simulink model "NataliaQAM16"  (Simulink 7.5)
settings: Solver=ode45  StartTime=0.0  StopTime=0.003  RelTol=1e-3
undefined symbols (not defined in the file or in its folder): CRC, Fs, get, Iter, Len, Max, sided, Two, Variance
libraries: dspobslib x6, commsequence2 x6, commblkintrlv2 x6, dspindex x5, commcnvcod2 x4, commcrc2 x2, commdigbbndam3 x2, dspsnks4 x2, dspxfrm3 x2, dspsigops x2, commseqgen2 x2, commutil2 x2
settings Model: Creator=Natalia  LastModifiedBy=Natalia

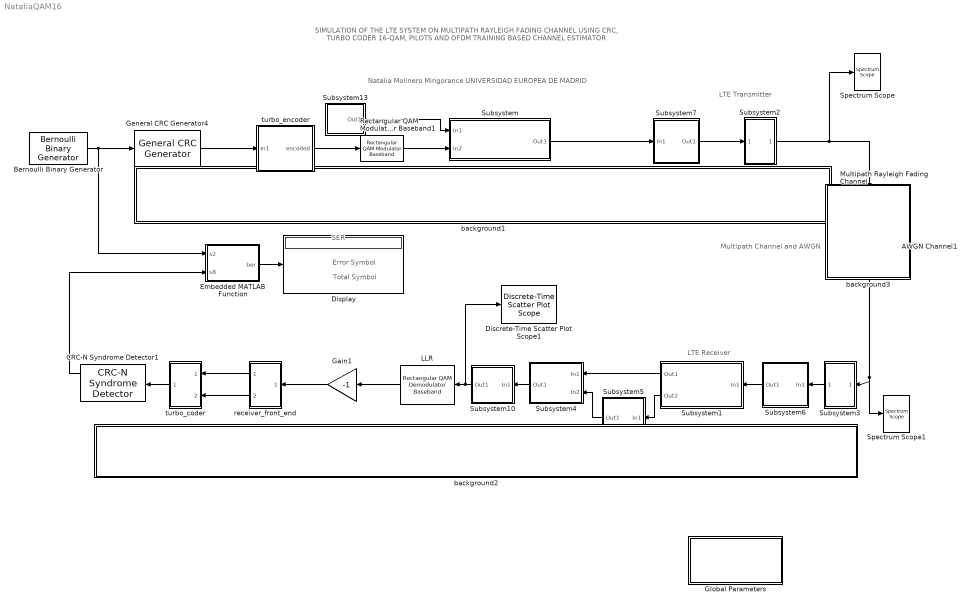
== system NataliaQAM16 ==
  note: SER
  note: Error Symbol
  note: Total Symbol
  note: SIMULATION OF THE LTE SYSTEM ON MULTIPATH RAYLEIGH FADING CHANNEL
      | USING CRC, TURBO CODER 16-QAM, PILOTS AND OFDM
      | TRAINING BASED CHANNEL ESTIMATOR
  note: Natalia Molinero Mingorance
      | UNIVERSIDAD EUROPEA DE MADRID
  note: LTE Transmitter
  note: LTE Receiver
  note: Multipath Channel
      | and AWGN
  AWGN Channel1 : commchan3/AWGN Channel  SystemSampleTime=-1  seed=32965  noiseMode="Signal to noise ratio  (Es/No)"  EbNodB=10  EsNodB=5  SNRdB=0  bitsPerSym=1  Ps=30/(5.5e5*11/15*2.4)*1.08  Tsym=80e-6  variance=1
  Bernoulli Binary Generator : commrandsrc2/Bernoulli Binary Generator  DialogController=commDDGCreate  DialogControllerArgs=DataTag0  SystemSampleTime=-1  P=0.5  seed=61  Ts=1  frameBased=on  sampPerFrame=20  orient=off  outDataType=boolean
  CRC-N Syndrome Detector1 : commcrc2/CRC-N Syndrome Detector  SystemSampleTime=-1  crcMethod=CRC-24  iniStates=[0]  numChecksums=1
  Discrete-Time Scatter Plot Scope1 : commsink2/Discrete-Time Scatter Plot Scope  Tag=ScatterPlot  SystemSampleTime=-1  sampPerSymb=1  offsetEye=0  numTraces=40  numNewFrames=10  LineMarkers=.  LineColors=b  fading=on  render=on  AxisGrid=on  xMin=-0.707933120701309  xMax=0.713103512853537  yMin=-0.710699489007895  yMax=0.71033714454695  inphaseLabel=In-phase Amplitude  quadratureLabel=Quadrature Amplitude  openScopeAtSimStart=on  FrameNumber=off  FigPos=get(0,'defaultfigureposition');  figTitle=Scatter Plot  numLinesMax=8  block_type_=scatter
  Display : Display
  Embedded MATLAB Function : Stateflow chart  TreatAsAtomicUnit=on
  Gain1 : Gain  Gain=-1  SaturateOnIntegerOverflow=on  OutDataTypeStr=Inherit: Same as input  ParamDataTypeStr=Inherit: Same as input
  General CRC Generator4 : commcrc2/General CRC Generator  genPoly=[24,23,6,5,1,0]  iniStates=[0]  numChecksums=1
  Global Parameters : Subsystem  mask(Global Parameters){EbNodB=11, Len=44, Iter=5, Seed=54123}
      mask prompts: EbNodB "Eb/No in dB:"; Len "Block size:"; Iter "Number of iterations:"
      mask help: Load global parameters in MATLAB workspace.
      mask init:
      | turbo_code_punc_setup;
      mask CallbackString: turbo_code_setup;|turbo_code_setup|turbo_code_setup;|turbo_code_setup;
      mask Display: disp(['Eb/No ' num2str(EbNodB,'%3.1f') 'dB'  sprintf('\n') 'Block size   ' num2str(Len,'%7.0f')  sprintf('\n') 'Iterations   ' num2str(Iter,'%3.0f')   sprintf('\n') 'Seed   ' num2str(Seed,'%7.0f')])
  LLR : commdigbbndam3/Rectangular QAM Demodulator Baseband  DialogController=commDDGCreate  DialogControllerArgs=DataTag1  M=16  PowType=Average Power  MinDist=2  AvgPow=0.5  PeakPow=1  Ph=0  Dec=Gray  Mapping=[0:15]  OutType=Bit  DecType=Log-likelihood ratio  VarSource=Dialog  Variance=Variance  outDtype1=double  outDtype2=double  derotateFactorWordLen=16  denormFactorWordLen=16  prodOutWordLen=32  prodOutRoundingMode=Floor  prodOutOverflowMode=Wrap  sumWordLen=32
  Multipath Rayleigh Fading Channel : commchan2/Multipath Rayleigh Fading Channel  SystemSampleTime=-1  Fd=299  simTs=8e-5/180  delayVec=[0 3e-6]  gainVecdB=[0 8]  normGain=on  Seed=936497248
  Rectangular QAM Modulator Baseband1 : commdigbbndam3/Rectangular QAM Modulator Baseband  DialogController=commDDGCreate  DialogControllerArgs=DataTag2  M=16  InType=Bit  Enc=Gray  Mapping=[0:15]  PowType=Average Power  MinDist=2  AvgPow=0.5  PeakPow=1  Ph=0  outDtype=double  outWordLen=16  outUDDataType=sfix(16)  outFracLenMode=Best precision  outFracLen=15
  Spectrum Scope : dspsnks4/Spectrum Scope  DialogController=dspdialog.SpectrumScope  DialogControllerArgs=DataTag3  SystemSampleTime=-1  ScopeProperties=on  Domain=Frequency  HorizSpan=1  UseBuffer=on  BufferSize=90  Overlap=64  inpFftLenInherit=on  FFTlength=1024  numAvg=16  DisplayProperties=off  AxisGrid=on  Memory=off  FrameNumber=on  AxisLegend=off  AxisZoom=off  OpenScopeAtSimStart=on  OpenScopeImmediately=off  FigPos=get(0,'defaultfigureposition')  AxisProperties=off  XUnits=Hertz  XRange=Two-sided ((-Fs/2...Fs/2])  XDisplay=0  InheritXIncr=on  XIncr=1.0  XLabel=Samples  XLimit=Auto  YUnits=dBW/Hertz  XMax=1  XMin=0  YLabel=Magnitude-squared, dB  LineProperties=off  wintypeSpecScope=Hann  RsSpecScope=50  betaSpecScope=5  winsampSpecScope=Periodic  XAxisParamsVer=6.9
      settings: YMin=-10  YMax=10
  Spectrum Scope1 : dspsnks4/Spectrum Scope  DialogController=dspdialog.SpectrumScope  DialogControllerArgs=DataTag4  SystemSampleTime=-1  ScopeProperties=on  Domain=Frequency  HorizSpan=1  UseBuffer=on  BufferSize=90  Overlap=64  inpFftLenInherit=on  FFTlength=1024  numAvg=16  DisplayProperties=off  AxisGrid=on  Memory=off  FrameNumber=on  AxisLegend=off  AxisZoom=off  OpenScopeAtSimStart=on  OpenScopeImmediately=off  FigPos=get(0,'defaultfigureposition')  AxisProperties=off  XUnits=Hertz  XRange=Two-sided ((-Fs/2...Fs/2])  XDisplay=0  InheritXIncr=on  XIncr=1.0  XLabel=Samples  XLimit=Auto  YUnits=dBW/Hertz  XMax=1  XMin=0  YLabel=Magnitude-squared, dB  LineProperties=off  wintypeSpecScope=Hann  RsSpecScope=50  betaSpecScope=5  winsampSpecScope=Periodic  XAxisParamsVer=6.9
      settings: YMin=-10  YMax=10
  Subsystem : Subsystem
      mask Display: disp('OFDM Baseband\nModulator\ndan\nAdd Cyclic Prefix')
  Subsystem1 : Subsystem
      mask Display: disp('OFDM Baseband\nDemodulator\ndan \nRemove Cyclic prefix')
  Subsystem10 : Subsystem
      mask Display: disp('Remove\nZero')
  Subsystem13 : Subsystem
      mask Display: disp('Training')
  Subsystem2 : Subsystem
      mask Display: disp('P/S')
  Subsystem3 : Subsystem
      mask Display: disp('S/P')
  Subsystem4 : Subsystem
      mask Display: disp('Channel\nCompensation')
  Subsystem5 : Subsystem
      mask Display: disp('Channel\nEstimator')
  Subsystem6 : Subsystem
      mask Display: disp('Training\nSeparation')
  Subsystem7 : Subsystem
      mask Display: disp('Training\nInsertion')
  background1 : Subsystem
      mask Display: disp('')
  background2 : Subsystem
      mask Display: disp('')
  background3 : Subsystem
      mask Display: disp('')
  receiver_front_end : Subsystem
  turbo_coder : Subsystem
  turbo_encoder : Subsystem
  wires:
  receiver_front_end/1(Out1) -> turbo_coder/1(In1)
  receiver_front_end/2(Out2) -> turbo_coder/2(In2)
  turbo_encoder/1(encoded) -> Rectangular QAM Modulator Baseband1/1
  LLR/1 -> Gain1/1
  Gain1/1 -> receiver_front_end/1(In1)
  Subsystem13/1(Out1) -> Subsystem/1(In1)
  Subsystem/1(Out1) -> Subsystem7/1(In1)
  Subsystem7/1(Out1) -> Subsystem2/1(In1)
  Rectangular QAM Modulator Baseband1/1 -> Subsystem/2(In2)
  Subsystem1/1(Out1) -> Subsystem4/1(In1)
  Subsystem1/2(Out2) -> Subsystem5/1(In1)
  Subsystem5/1(Out1) -> Subsystem4/2(In2)
  Subsystem4/1(Out1) -> Subsystem10/1(In1)
  Subsystem6/1(Out1) -> Subsystem1/1(In1)
  Subsystem3/1(Out1) -> Subsystem6/1(In1)
  Subsystem10/1(Out1) -> LLR/1, Discrete-Time Scatter Plot Scope1/1
  Multipath Rayleigh Fading Channel/1 -> AWGN Channel1/1
  AWGN Channel1/1 -> Subsystem3/1(In1), Spectrum Scope1/1
  Subsystem2/1(Out1) -> Multipath Rayleigh Fading Channel/1, Spectrum Scope/1
  General CRC Generator4/1 -> turbo_encoder/1(In1)
  turbo_coder/1(Out1) -> CRC-N Syndrome Detector1/1
  Embedded MATLAB Function/1(ber) -> Display/1
  Bernoulli Binary Generator/1 -> General CRC Generator4/1, Embedded MATLAB Function/1(s2)
  CRC-N Syndrome Detector1/1 -> Embedded MATLAB Function/2(s8)

== system NataliaQAM16/Global Parameters ==

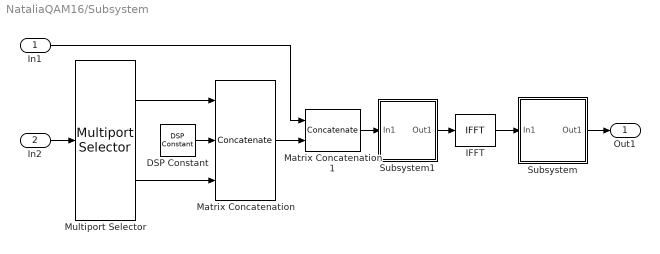
== system NataliaQAM16/Subsystem ==
  In1 : Inport  OutDataType=sfix(16)  OutScaling=2^0
  In2 : Inport  Port=2  OutDataType=sfix(16)  OutScaling=2^0
  DSP Constant : dspobslib/DSP Constant  SystemSampleTime=-1  Value=0  SampleMode=Discrete  discreteOutput=Frame-based  continuousOutput=Sample-based  sampTime=16e-5/2  framePeriod=16e-5/2  dataType=Inherit from 'Constant value'  isSigned=on  wordLen=16  udDataType=sfix(16)  fracBitsMode=Best precision  numFracBits=15  InterpretAs1D=off  Ts=16e-5/2  FramebasedOutput=on
  IFFT : dspxfrm3/IFFT  DialogController=dspDDGCreate  DialogControllerArgs=DataTag5  CompMethod=Table lookup  TableOpt=HYBRID  TableOptActive=Speed  BitRevOrder=off  cs_in=off  SkipNorm=on  InheritFFTLength=on  FFTLength=64  mode=Real  outSamplingMode=Frame based  firstCoeffDataTypeStr=Inherit: Same word length as input  firstCoeffLastDataTypeStr=Inherit: Same word length as input  outputMin=[]  outputMax=[]  roundingMode=Floor  overflowMode=off
  Matrix Concatenation : Concatenate  NumInputs=3  Mode=Multidimensional array
  Matrix Concatenation1 : Concatenate  Mode=Multidimensional array  ConcatenateDimension=2
  Multiport Selector : dspindex/Multiport Selector  rowsOrCols=Rows  idxCellArray={1:11,12:22}  idxErrMode=Clip Index
  Subsystem : Subsystem
      mask Display: disp('Add\nCyclic Prefix')
  Subsystem1 : Subsystem
      mask Display: disp('Zero Pad')
  Out1 : Outport
  wires:
  IFFT/1 -> Subsystem/1(In1)
  Multiport Selector/1 -> Matrix Concatenation/1
  Multiport Selector/2 -> Matrix Concatenation/3
  DSP Constant/1 -> Matrix Concatenation/2
  Subsystem1/1(Out1) -> IFFT/1
  Subsystem/1(Out1) -> Out1/1
  In2/1 -> Multiport Selector/1
  Matrix Concatenation1/1 -> Subsystem1/1(In1)
  Matrix Concatenation/1 -> Matrix Concatenation1/2
  In1/1 -> Matrix Concatenation1/1

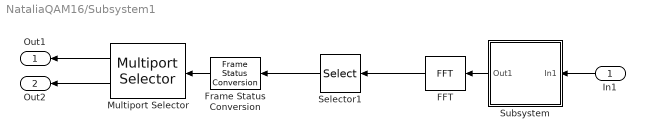
== system NataliaQAM16/Subsystem1 ==
  In1 : Inport  OutDataType=sfix(16)  OutScaling=2^0
  FFT : dspxfrm3/FFT  DialogController=dspDDGCreate  DialogControllerArgs=DataTag6  CompMethod=Table lookup  TableOpt=HYBRID  TableOptActive=Speed  BitRevOrder=off  InheritFFTLength=on  FFTLength=64  SkipNorm=on  firstCoeffDataTypeStr=Inherit: Same word length as input  firstCoeffLastDataTypeStr=Inherit: Same word length as input  outputMin=[]  outputMax=[]  roundingMode=Floor  overflowMode=off
  Frame Status Conversion : dspobslib/Frame Status Conversion  SystemSampleTime=-1  growRefPort=off  outframe=Frame-based
  Multiport Selector : dspindex/Multiport Selector  rowsOrCols=Columns  idxCellArray={1,2}  idxErrMode=Clip Index
  Selector1 : Selector  NumberOfDimensions=2  InputPortWidth=64  IndexOptions=Index vector (dialog),Select all  Indices=[54:64,1:12],-1  OutputSizes=1
  Subsystem : Subsystem
      mask Display: disp('Remove\nCyclic Prefix')
  Out1 : Outport
  Out2 : Outport  Port=2
  wires:
  FFT/1 -> Selector1/1
  Selector1/1 -> Frame Status Conversion/1
  Subsystem/1(Out1) -> FFT/1
  In1/1 -> Subsystem/1(In1)
  Frame Status Conversion/1 -> Multiport Selector/1
  Multiport Selector/1 -> Out1/1
  Multiport Selector/2 -> Out2/1

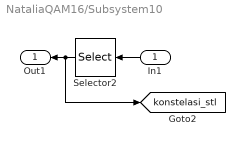
== system NataliaQAM16/Subsystem10 ==
  In1 : Inport  OutDataType=sfix(16)  OutScaling=2^0
  Selector2 : Selector  NumberOfDimensions=2  InputPortWidth=31  IndexOptions=Index vector (dialog),Select all  Indices=[1:11,13:23],-1  OutputSizes=1
  Out1 : Outport
  tag scope: konstelasi_stl=global
  wires:
  Selector2/1 -> Out1/1, [konstelasi_stl]
  In1/1 -> Selector2/1

== system NataliaQAM16/Subsystem13 ==
  PN Sequence Generator : commseqgen2/PN Sequence Generator  poly=[1 0 0 0 0 1 1]  ini_sta=[0 0 0 0 0 1]  outBitMaskSource=Dialog parameter  shift=0  Ts=16e-5/2/23  frameBased=on  sampPerFrame=23  reset=off  bitPackedOutputs=off  outDataType=double  numPackedBits=8  bitPackDataSigned=off  bitPackedOutDType=double
  Unipolar to Bipolar Converter : commutil2/Unipolar to Bipolar Converter  SystemSampleTime=-1  M=2  polarity=Positive  dataType=Inherit via internal rule
  Out1 : Outport
  wires:
  PN Sequence Generator/1 -> Unipolar to Bipolar Converter/1
  Unipolar to Bipolar Converter/1 -> Out1/1

== system NataliaQAM16/Subsystem2 ==
  In1 : Inport  OutDataType=sfix(16)  OutScaling=2^0
  Unbuffer3 : dspbuff3/Unbuffer  ic=0
  Out1 : Outport
  wires:
  In1/1 -> Unbuffer3/1
  Unbuffer3/1 -> Out1/1

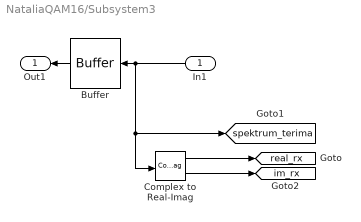
== system NataliaQAM16/Subsystem3 ==
  In1 : Inport  OutDataType=sfix(16)  OutScaling=2^0
  Buffer : dspbuff3/Buffer  N=180  V=0  ic=0
  Complex to Real-Imag : ComplexToRealImag
  Out1 : Outport
  tag scope: im_rx=global, real_rx=global, spektrum_terima=global
  wires:
  In1/1 -> Buffer/1, [spektrum_terima], Complex to Real-Imag/1
  Buffer/1 -> Out1/1
  Complex to Real-Imag/1 -> [real_rx]
  Complex to Real-Imag/2 -> [im_rx]

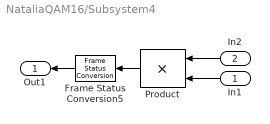
== system NataliaQAM16/Subsystem4 ==
  In1 : Inport  OutDataType=sfix(16)  OutScaling=2^0
  In2 : Inport  Port=2  OutDataType=sfix(16)  OutScaling=2^0
  Frame Status Conversion5 : dspobslib/Frame Status Conversion  SystemSampleTime=-1  growRefPort=off  outframe=Frame-based
  Product : Product  OutDataType=sfix(16)  OutScaling=2^0  SaturateOnIntegerOverflow=on  OutDataTypeStr=Inherit: Same as first input
  Out1 : Outport
  wires:
  Product/1 -> Frame Status Conversion5/1
  Frame Status Conversion5/1 -> Out1/1
  In2/1 -> Product/1
  In1/1 -> Product/2

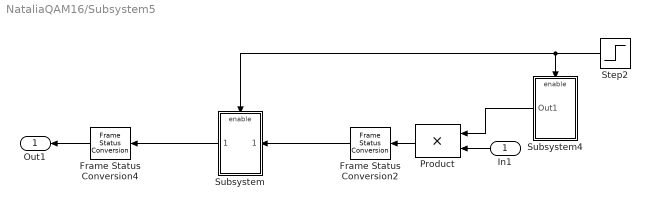
== system NataliaQAM16/Subsystem5 ==
  In1 : Inport  OutDataType=sfix(16)  OutScaling=2^0
  Frame Status Conversion2 : dspobslib/Frame Status Conversion  SystemSampleTime=-1  growRefPort=off  outframe=Frame-based
  Frame Status Conversion4 : dspobslib/Frame Status Conversion  SystemSampleTime=-1  growRefPort=off  outframe=Frame-based
  Product : Product  OutDataType=sfix(16)  OutScaling=2^0  SaturateOnIntegerOverflow=on  OutDataTypeStr=Inherit: Same as first input
  Step2 : Step  Time=16e-5/2  SampleTime=16e-5/2
  Subsystem : Subsystem
  Subsystem4 : Subsystem  TreatAsAtomicUnit=on
  Out1 : Outport
  wires:
  Step2/1 -> Subsystem4/Enable, Subsystem/Enable
  Subsystem4/1(Out1) -> Product/1
  Product/1 -> Frame Status Conversion2/1
  Frame Status Conversion2/1 -> Subsystem/1(In1)
  Frame Status Conversion4/1 -> Out1/1
  In1/1 -> Product/2
  Subsystem/1(Out1) -> Frame Status Conversion4/1

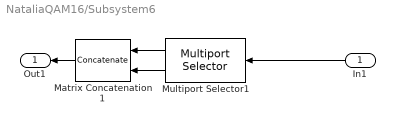
== system NataliaQAM16/Subsystem6 ==
  In1 : Inport  OutDataType=sfix(16)  OutScaling=2^0
  Matrix Concatenation1 : Concatenate  Mode=Multidimensional array  ConcatenateDimension=2
  Multiport Selector1 : dspindex/Multiport Selector  rowsOrCols=Rows  idxCellArray={91:180,1:90}  idxErrMode=Clip Index
  Out1 : Outport
  wires:
  Multiport Selector1/2 -> Matrix Concatenation1/2
  Multiport Selector1/1 -> Matrix Concatenation1/1
  In1/1 -> Multiport Selector1/1
  Matrix Concatenation1/1 -> Out1/1

== system NataliaQAM16/Subsystem7 ==
  In1 : Inport  OutDataType=sfix(16)  OutScaling=2^0
  Matrix Concatenation : Concatenate  Mode=Multidimensional array
  Multiport Selector : dspindex/Multiport Selector  rowsOrCols=Columns  idxCellArray={1,2}  idxErrMode=Clip Index
  Out1 : Outport
  wires:
  Multiport Selector/1 -> Matrix Concatenation/1
  Multiport Selector/2 -> Matrix Concatenation/2
  In1/1 -> Multiport Selector/1
  Matrix Concatenation/1 -> Out1/1

== system NataliaQAM16/background1 ==

== system NataliaQAM16/background2 ==

== system NataliaQAM16/background3 ==

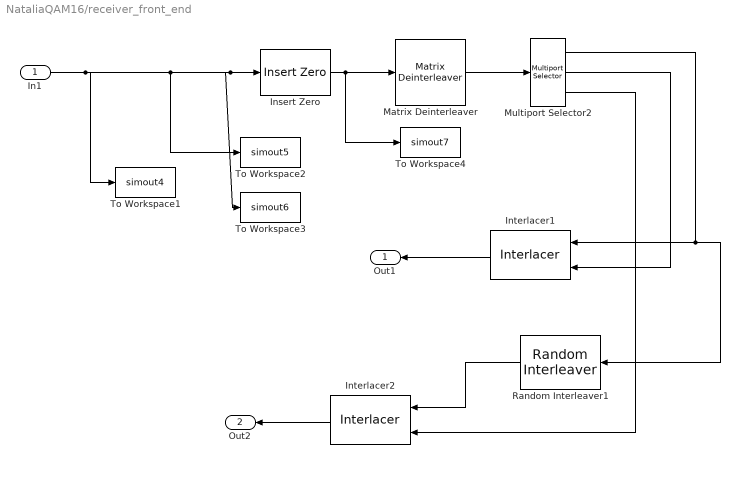
== system NataliaQAM16/receiver_front_end ==
  In1 : Inport
  Insert Zero : commsequence2/Insert Zero  insertZeroVector=[1 1 0 1 0 1].'
  Interlacer1 : commsequence2/Interlacer
  Interlacer2 : commsequence2/Interlacer
  Matrix Deinterleaver : commblkintrlv2/Matrix Deinterleaver  SystemSampleTime=-1  Nrows=3  Ncols=44
  Multiport Selector2 : dspindex/Multiport Selector  rowsOrCols=Rows  idxCellArray={1:Len, Len+1:2*Len, 2*Len+1:3*Len}  idxErrMode=Clip Index
  Random Interleaver1 : commblkintrlv2/Random Interleaver  SystemSampleTime=-1  N=Len  seed=Seed
  To Workspace1 : ToWorkspace  VariableName=simout4  SampleTime=-1  SaveFormat=Array
  To Workspace2 : ToWorkspace  VariableName=simout5  SampleTime=-1  SaveFormat=Array
  To Workspace3 : ToWorkspace  VariableName=simout6  SampleTime=-1  SaveFormat=Array
  To Workspace4 : ToWorkspace  VariableName=simout7  SampleTime=-1  SaveFormat=Array
  Out1 : Outport
  Out2 : Outport  Port=2
  wires:
  Multiport Selector2/1 -> Interlacer1/1, Random Interleaver1/1
  Multiport Selector2/2 -> Interlacer1/2
  Random Interleaver1/1 -> Interlacer2/1
  Multiport Selector2/3 -> Interlacer2/2
  In1/1 -> To Workspace1/1, To Workspace2/1, Insert Zero/1, To Workspace3/1
  Interlacer1/1 -> Out1/1
  Interlacer2/1 -> Out2/1
  Matrix Deinterleaver/1 -> Multiport Selector2/1
  Insert Zero/1 -> Matrix Deinterleaver/1, To Workspace4/1

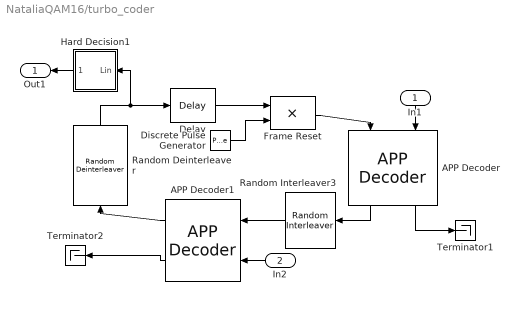
== system NataliaQAM16/turbo_coder ==
  In1 : Inport
  In2 : Inport  Port=2
  APP Decoder : commcnvcod2/APP Decoder  trellis=trellis  termMethod=Truncated  algorithm=Max*  maxStarNumScaleBits=3
  APP Decoder1 : commcnvcod2/APP Decoder  trellis=trellis  termMethod=Truncated  algorithm=Max*  maxStarNumScaleBits=3
  Delay : dspsigops/Delay  dly_unit=Samples  delay=Len  ic_detail=off  dif_ic_for_ch=off  dif_ic_for_dly=off  ic=0  reset_popup=None
  Discrete Pulse Generator : DiscretePulseGenerator  Amplitude=1  Period=Iter  PulseWidth=Iter-1  PhaseDelay=1  SampleTime=1
  Frame Reset : Product  SaturateOnIntegerOverflow=on  InputSameDT=on  OutDataTypeStr=Inherit: Same as first input
  Hard Decision1 : Subsystem
      mask Type: Hard Decision
      mask Description: Likelihood to binary transformation.
  Random Deinterleaver : commblkintrlv2/Random Deinterleaver  SystemSampleTime=-1  N=Len  seed=Seed
  Random Interleaver3 : commblkintrlv2/Random Interleaver  SystemSampleTime=-1  N=Len  seed=Seed
  Terminator1 : Terminator
  Terminator2 : Terminator
  Out1 : Outport
  wires:
  APP Decoder1/1 -> Random Deinterleaver/1
  APP Decoder/2 -> Terminator1/1
  APP Decoder1/2 -> Terminator2/1
  Random Deinterleaver/1 -> Delay/1, Hard Decision1/1(Lin)
  Random Interleaver3/1 -> APP Decoder1/1
  APP Decoder/1 -> Random Interleaver3/1
  Frame Reset/1 -> APP Decoder/1
  Delay/1 -> Frame Reset/1
  Discrete Pulse Generator/1 -> Frame Reset/2
  Hard Decision1/1(0/1) -> Out1/1
  In1/1 -> APP Decoder/2
  In2/1 -> APP Decoder1/2

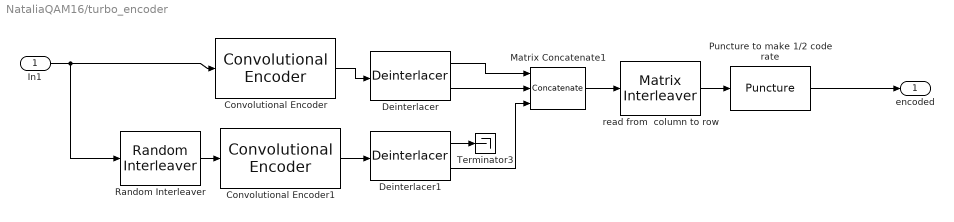
== system NataliaQAM16/turbo_encoder ==
  In1 : Inport
  Convolutional Encoder : commcnvcod2/Convolutional Encoder  trellis=trellis  opMode=Continuous  hasIniStPort=off  hasFinStPort=off  usePuncVector=off  punctureVector=[ 1 1 0 1 0 1]'  reset=Unused parameter value
  Convolutional Encoder1 : commcnvcod2/Convolutional Encoder  trellis=trellis  opMode=Truncated (reset every frame)  hasIniStPort=off  hasFinStPort=off  usePuncVector=off  punctureVector=[ 1 1 0 1 0 1]'  reset=Unused parameter value
  Deinterlacer : commsequence2/Deinterlacer
  Deinterlacer1 : commsequence2/Deinterlacer
  Matrix Concatenate1 : Concatenate  NumInputs=3  Mode=Multidimensional array
  Puncture to make 1/2 code rate : commsequence2/Puncture  punctureVector=[1 1 0 1 0 1].'
  Random Interleaver : commblkintrlv2/Random Interleaver  SystemSampleTime=-1  N=Len  seed=Seed
  Terminator3 : Terminator
  read from  column to row : commblkintrlv2/Matrix Interleaver  SystemSampleTime=-1  Nrows=3  Ncols=Len
  encoded : Outport
  wires:
  In1/1 -> Convolutional Encoder/1, Random Interleaver/1
  Puncture to make 1/2 code rate/1 -> encoded/1
  Random Interleaver/1 -> Convolutional Encoder1/1
  Convolutional Encoder/1 -> Deinterlacer/1
  Convolutional Encoder1/1 -> Deinterlacer1/1
  Deinterlacer1/1 -> Terminator3/1
  Deinterlacer/1 -> Matrix Concatenate1/1
  Deinterlacer1/2 -> Matrix Concatenate1/3
  read from  column to row/1 -> Puncture to make 1/2 code rate/1
  Matrix Concatenate1/1 -> read from  column to row/1
  Deinterlacer/2 -> Matrix Concatenate1/2

== system NataliaQAM16/Subsystem/Subsystem ==
  In1 : Inport  OutDataType=sfix(16)  OutScaling=2^0
  Selector3 : Selector  NumberOfDimensions=2  InputPortWidth=64  IndexOptions=Index vector (dialog),Select all  Indices=[39:64,1:64],-1  OutputSizes=1
  Out1 : Outport
  wires:
  Selector3/1 -> Out1/1
  In1/1 -> Selector3/1

== system NataliaQAM16/Subsystem/Subsystem1 ==
  In1 : Inport  OutDataType=sfix(16)  OutScaling=2^0
  Selector : Selector  NumberOfDimensions=2  InputPortWidth=64  IndexOptions=Index vector (dialog),Select all  Indices=[12:64,1:11],-1  OutputSizes=1
  Zero Pad : dspsigops/Pad  padAlong=Columns and rows  dimsToPad=1  valSrc=Specify via dialog  padVal=0  spec=Output size  padNumOutRowsSpecMethod=User-specified  numOutRows=64  padNumOutColsSpecMethod=User-specified  numOutCols=2  isVarDimsMode=off  padBeginning=0  padEnd=0  outSizeMode=User-specified  outSize=1  padSigAt=End  trunc_flag=None  roundingMode=Floor  overflowMode=off  truncOrWrapMode=Truncate  wrap_flag=None
  Out1 : Outport
  wires:
  Zero Pad/1 -> Selector/1
  In1/1 -> Zero Pad/1
  Selector/1 -> Out1/1

== system NataliaQAM16/Subsystem1/Subsystem ==
  In1 : Inport  OutDataType=sfix(16)  OutScaling=2^0
  Selector4 : Selector  NumberOfDimensions=2  InputPortWidth=78  IndexOptions=Index vector (dialog),Select all  Indices=[27:90],-1  OutputSizes=1
  Out1 : Outport
  wires:
  Selector4/1 -> Out1/1
  In1/1 -> Selector4/1

== system NataliaQAM16/Subsystem5/Subsystem ==
  In1 : Inport  OutDataType=sfix(16)  OutScaling=2^0
  Enable : EnablePort
  Math Function : Math  Operator=reciprocal  SaturateOnIntegerOverflow=on
  Out1 : Outport
  wires:
  In1/1 -> Math Function/1
  Math Function/1 -> Out1/1

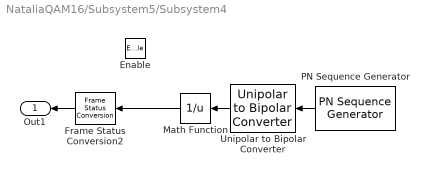
== system NataliaQAM16/Subsystem5/Subsystem4 ==
  Enable : EnablePort
  Frame Status Conversion2 : dspobslib/Frame Status Conversion  SystemSampleTime=-1  growRefPort=off  outframe=Frame-based
  Math Function : Math  Operator=reciprocal  SaturateOnIntegerOverflow=on
  PN Sequence Generator : commseqgen2/PN Sequence Generator  poly=[1 0 0 0 0 1 1]  ini_sta=[0 0 0 0 0 1]  outBitMaskSource=Dialog parameter  shift=0  Ts=16e-5/2/23  frameBased=on  sampPerFrame=23  reset=off  bitPackedOutputs=off  outDataType=double  numPackedBits=8  bitPackDataSigned=off  bitPackedOutDType=double
  Unipolar to Bipolar Converter : commutil2/Unipolar to Bipolar Converter  SystemSampleTime=-1  M=2  polarity=Positive  dataType=Inherit via internal rule
  Out1 : Outport
  wires:
  PN Sequence Generator/1 -> Unipolar to Bipolar Converter/1
  Frame Status Conversion2/1 -> Out1/1
  Math Function/1 -> Frame Status Conversion2/1
  Unipolar to Bipolar Converter/1 -> Math Function/1

== system NataliaQAM16/turbo_coder/Hard Decision1 ==
  Lin : Inport
  Constant : Constant  Value=0
  Relational Operator : RelationalOperator  InputSameDT=on
  0/1 : Outport
  wires:
  Constant/1 -> Relational Operator/2
  Lin/1 -> Relational Operator/1
  Relational Operator/1 -> 0/1/1

== matlab function Embedded MATLAB Function ==
  data: s2 input double; ber output double; s8 input double
function ber = fcn(s2,s8)
y=s2-s8;
z=0;
for i=1:20
    if y(i)~=0
        z=z+1;
    end
    
end
ber=z/(length(s2)*38);
